simulink model "Ilian_Boost"  (R2018a)
settings: Solver=VariableStepAuto  StartTime=0.0  StopTime=0.2  RelTol=1e-3
libraries: powerlib x11
settings Model: Creator=Ilian  LastModifiedBy=ivank

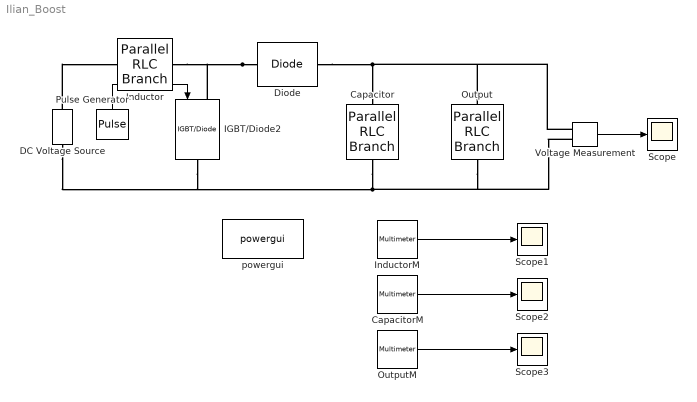
== system Ilian_Boost ==
  Capacitor : powerlib/Elements/Parallel RLC Branch  LConnTagsString=a  RConnTagsString=__new0  BranchType=C  Resistance=0  Inductance=1e-3  SetiL0=off  InitialCurrent=0  Capacitance=3.46e-6  Setx0=off  InitialVoltage=0  Measurements=Branch voltage and current
  CapacitorM : powerlib/Measurements/Multimeter  PhasorSimulation=off  OutputType=Complex  sel=[1 4]  L=6  Gain=[1 1]  yselected={'Ub: Capacitor','Ib: Capacitor'};  PSBOutputType=1  PSBequivalent=0  AxesSetting=[0,0.1,-100,100]  Display=1  SavedBlockNames=-11
  DC Voltage Source : powerlib/Electrical Sources/DC Voltage Source  Amplitude=12  Measurements=None
  Diode : powerlib/Power Electronics/Diode  Ron=0.001  Lon=0  Vf=0.8  IC=0  UseSnubber=0  Rs=500  Cs=250e-9  Measurements=off
  IGBT/Diode2 : powerlib/Power Electronics/IGBT//Diode  Ron=1e-3  Rs=1e5  Cs=inf  Measurements=off
  Inductor : powerlib/Elements/Parallel RLC Branch  LConnTagsString=a  RConnTagsString=__new0  BranchType=L  Resistance=0  Inductance=21.675e-3  SetiL0=off  InitialCurrent=0  Capacitance=0  Setx0=off  InitialVoltage=0  Measurements=Branch voltage and current
  "InductorM " : powerlib/Measurements/Multimeter  PhasorSimulation=off  OutputType=Complex  sel=[2 5]  L=6  Gain=[1 1]  yselected={'Ub: Inductor','Ib: Inductor'};  PSBOutputType=1  PSBequivalent=0  AxesSetting=[0,0.1,-100,100]  Display=1  SavedBlockNames=-11
  Output : powerlib/Elements/Parallel RLC Branch  LConnTagsString=a  RConnTagsString=__new0  BranchType=R  Resistance=7.225  Inductance=1e-3  SetiL0=off  InitialCurrent=0  Capacitance=100*10e-6  Setx0=off  InitialVoltage=0  Measurements=Branch voltage and current
  OutputM : powerlib/Measurements/Multimeter  PhasorSimulation=off  OutputType=Complex  sel=[3 6]  L=6  Gain=[1 1]  yselected={'Ub: Output','Ib: Output'};  PSBOutputType=1  PSBequivalent=0  AxesSetting=[0,0.1,-100,100]  Display=1  SavedBlockNames=-11
  Pulse Generator : DiscretePulseGenerator  PulseType=Time based  Amplitude=5  Period=1/5000  PulseWidth=85
  Scope{,1..3} (4 alike) : Scope
  Voltage Measurement : powerlib/Measurements/Voltage Measurement  PhasorSimulation=off  OutputType=Complex  PSBequivalent=0
  powergui : powerlib/powergui  Priority=1  SimulationMode=Continuous  SampleTime=50e-6  frequency=60  Iterations=50  frequencyindice=0  Pbase=100e6  ErrMax=1e-4  UnitsV=kV  UnitsW=MW  buscounter=0  FunctionMessages=off  echomessages=off  EnableUseOfTLC=off  CurrentSourceSwitches=off  DisableSnubberDevices=off  DisableRonSwitches=off  DisableVfSwitches=off  DisplayEquations=off  SolverType=Tustin/Backward Euler (TBE)  Interpol=off  ExternalGateDelay=off  methode=off  Ts=100  x0status=blocks  SPID=on  SwTol=0  HookPort=off  RestoreLinks=warning  ResistiveCurrentMeasurement=off  Frange=[0:2:500]  Ylog=off  Xlog=on  ShowGrid=off  save=off  variable=ZData  structure=0  ZoomFFT=off  StartTime=0.0  cycles=1  DisplayStyle=1  fundamental=60  FreqAxis=off  MaxFrequency=1000  frequencyindicesteady=1  RmsSteady=1  display=off
  wires:
  Voltage Measurement/1 -> Scope/1
  "InductorM "/1 -> Scope1/1
  Pulse Generator/1 -> IGBT/Diode2/1
  CapacitorM/1 -> Scope2/1
  OutputM/1 -> Scope3/1
  connections:
  Diode/LConn1 -- Inductor/RConn1 -- IGBT/Diode2/LConn1
  Capacitor/RConn1 -- DC Voltage Source/LConn1 -- IGBT/Diode2/RConn1 -- Voltage Measurement/LConn2 -- Output/RConn1
  Diode/RConn1 -- Output/LConn1 -- Voltage Measurement/LConn1 -- Capacitor/LConn1
  DC Voltage Source/RConn1 -- Inductor/LConn1
